simulink model "module_buck"  (R2014a)
settings: Solver=ode45  StartTime=0.0  StopTime=.001  MaxStep=0.1e-6  RelTol=1e-3
values from neighbouring files (symbols this model uses):
  A1simple = [a1,                               a3,       0,                  0,                              0 ... (first row only)    [array_init.m]
  B1 = [B1top; B1bot]    [array_init.m]
  B2 = [0; 0; Vref*b1; Vref*b2; Vref*b3]    [array_init.m]
  x0 = [0;1.8;0;0;0]    [array_init.m]
undefined symbols (not defined in the file or in its folder): fs
libraries: simulink x1
settings Model: Creator=Dragan Maksimovic  LastModifiedBy=Taylor
settings DataIOCC: SignalLogging=off  DSMLogging=off
settings OptimizationCC: InlineParams=on  ExpressionDepthLimit=2147483647
settings DebuggingCC: UnderspecifiedInitializationDetection=Classic  FcnCallInpInsideContextMsg=UseLocalSettings  StateNameClashWarn=warning
settings GRTTargetCC: CombineOutputUpdateFcns=off  GRTInterface=on

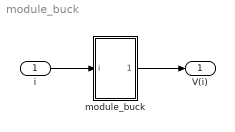
== system module_buck ==
  i : Inport
  module_buck : Subsystem
  V(i) : Outport
  wires:
  module_buck/1(Out2) -> V(i)/1
  i/1 -> module_buck/1(i)

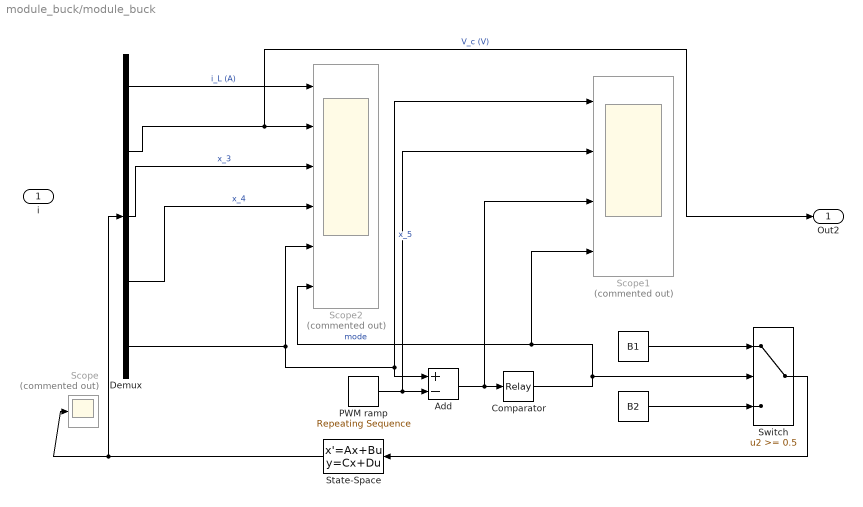
== system module_buck/module_buck ==
  i : Inport
  " " : Constant  Value=B2  VectorParams1D=off
  " " : Constant  Value=B1  VectorParams1D=off
  Add : Sum  Inputs=+-
  Comparator : Relay  OnSwitchValue=0  OffSwitchValue=0
  Demux : Demux  Outputs=5
  PWM ramp : simulink/Sources/Repeating Sequence  rep_seq_t=[0 1/fs]  rep_seq_y=[0 1]
  Scope : Scope  Commented=on
  Scope1 : Scope  Commented=on  NumInputPorts=4
      settings: ShowLegends=on  TimeRange=3.000131492439188e-05  YMin=1.74~-5~-5~-5  YMax=1.84~10~5~5
  Scope2 : Scope  Commented=on  NumInputPorts=6
      settings: ShowLegends=on  TimeRange=3.000131492439188e-05  YMin=0.5~1.988~0.0085~-0.0025~0.945~0  YMax=3.5~1.992~0.01175~0.0225~0.98~1  SaveName=ScopeData2
  State-Space : StateSpace  A=A1simple  B=eye(5)  C=eye(5)  D=zeros(5)  X0=x0
  Switch : Switch  Threshold=0.5
  Out2 : Outport
  wires:
  Demux/4 -> Scope2/4  "x_4"
  Switch/1 -> State-Space/1
  " "/1 -> Switch/3
  Add/1 -> Comparator/1, Scope1/3
  " "/1 -> Switch/1
  Demux/5 -> Scope1/1, Add/1, Scope2/5  "x_5"
  PWM ramp/1 -> Add/2, Scope1/2
  Comparator/1 -> Switch/2, Scope2/6, Scope1/4  "mode"
  Demux/3 -> Scope2/3  "x_3"
  Demux/1 -> Scope2/1  "i_L (A)"
  State-Space/1 -> Demux/1, Scope/1
  Demux/2 -> Scope2/2, Out2/1  "V_c (V)"
